simulink model "realtime"  (R2024b)
settings: Solver=VariableStepAuto  StartTime=0.0  StopTime=10.0  RelTol=1e-3
values from neighbouring files (symbols this model uses):
  C = Tc/(Tc+Ts)    [Observer_and_complementary_filter.m]    (also in init.m = @(q) [)
undefined symbols (not defined in the file or in its folder): denH, denHw, DiscIntNeverNeededParam, drv, dspblkCoreblockFVToolHelper, gbox, gcbh, integral, numH, numHw, sens, Ts, wheel
settings Model: Creator=lucag  LastModifiedBy=lucag

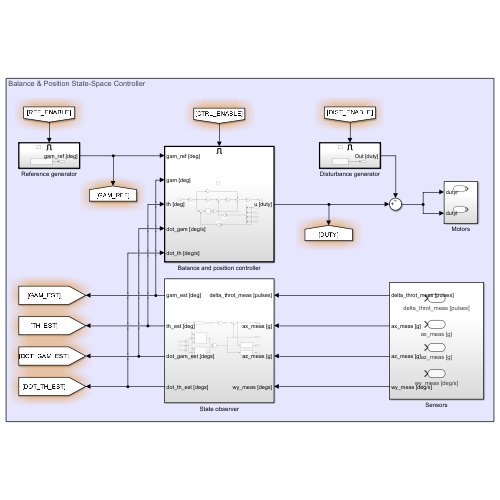
[thumbnail: Simulink's stored preview of the top-level diagram]
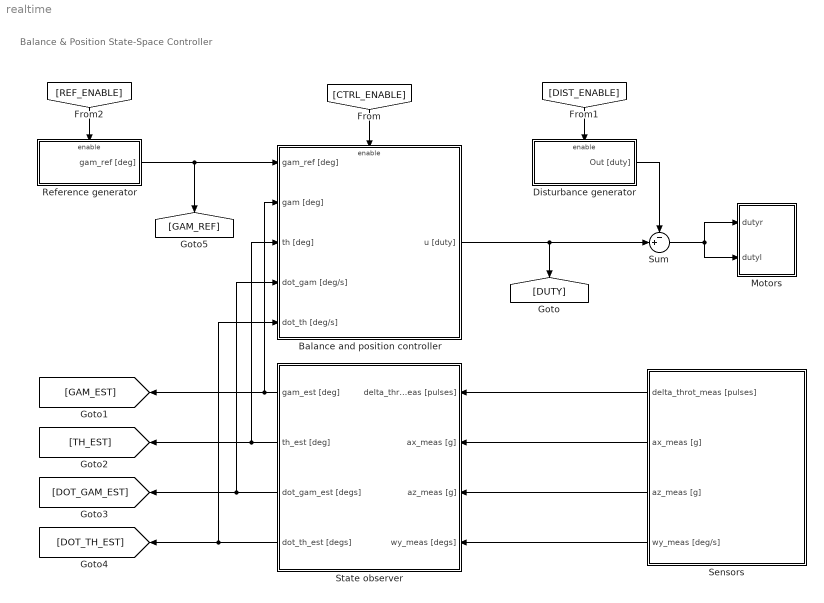
== system realtime ==
  note: Balance & Position State-Space Controller
  Balance and position controller : Subsystem  TreatAsAtomicUnit=on
  Disturbance generator : Subsystem  TreatAsAtomicUnit=on
  Motors : Subsystem
  Reference generator : Subsystem  TreatAsAtomicUnit=on
  Sensors : Subsystem
  State observer : Subsystem
  Sum : Sum  Inputs=-+|
  wires:
  [CTRL_ENABLE] -> Balance and position controller/Enable
  Balance and position controller/1(u [duty]) -> Sum/2, [DUTY]
  Disturbance generator/1(Out [duty]) -> Sum/1
  [DIST_ENABLE] -> Disturbance generator/Enable
  Sum/1 -> Motors/2(dutyl), Motors/1(dutyr)
  Sensors/1(delta_throt_meas [pulses]) -> State observer/1(delta_throt_meas [pulses])
  Sensors/2(ax_meas [g]) -> State observer/2(ax_meas [g])
  Sensors/3(az_meas [g]) -> State observer/3(az_meas [g])
  Sensors/4(wy_meas [deg/s]) -> State observer/4(wy_meas [degs])
  State observer/1(gam_est [deg]) -> [GAM_EST], Balance and position controller/2(gam [deg])
  State observer/2(th_est [deg]) -> [TH_EST], Balance and position controller/3(th [deg])
  State observer/3(dot_gam_est [degs]) -> Balance and position controller/4(dot_gam [deg/s]), [DOT_GAM_EST]
  State observer/4(dot_th_est [degs]) -> Balance and position controller/5(dot_th [deg/s]), [DOT_TH_EST]
  Reference generator/1(gam_ref [deg]) -> Balance and position controller/1(gam_ref [deg]), [GAM_REF]
  [REF_ENABLE] -> Reference generator/Enable

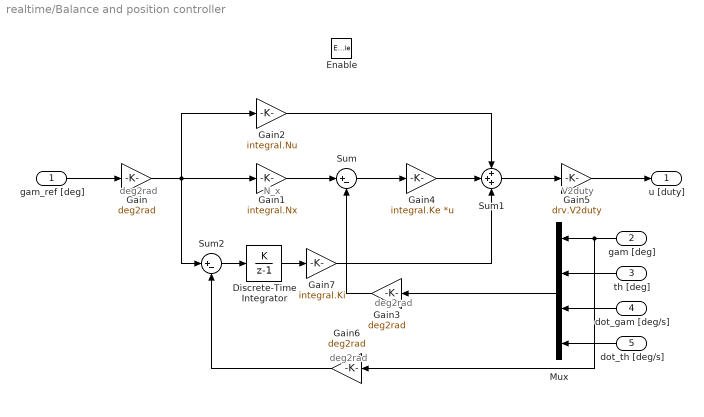
== system realtime/Balance and position controller ==
  note: deg2rad
  note: N_x
  note: V2duty
  note: deg2rad
  note: deg2rad
  gam_ref [deg] : Inport
  gam [deg] : Inport  Port=2
  th [deg] : Inport  Port=3
  dot_gam [deg/s] : Inport  Port=4
  dot_th [deg/s] : Inport  Port=5
  Enable : EnablePort
  Discrete-Time Integrator : DiscreteIntegrator  IntegratorMethod=Accumulation: Forward Euler  SampleTime=Ts  ICPrevOutput=DiscIntNeverNeededParam  ICPrevScaledInput=DiscIntNeverNeededParam
  Gain : Gain  Gain=deg2rad
  Gain1 : Gain  Gain=integral.Nx
  Gain2 : Gain  Gain=integral.Nu
  Gain3 : Gain  Gain=deg2rad
  Gain4 : Gain  Gain=integral.Ke  Multiplication=Matrix(K*u)
  Gain5 : Gain  Gain=drv.V2duty
  Gain6 : Gain  Gain=deg2rad
  Gain7 : Gain  Gain=integral.Ki
  Mux : Mux
  Sum : Sum  Inputs=|+-
  Sum1 : Sum  Inputs=+++
  Sum2 : Sum  Inputs=|+-
  u [duty] : Outport
  wires:
  dot_th [deg/s]/1 -> Mux/4
  Gain/1 -> Sum2/1, Gain2/1, Gain1/1
  Sum/1 -> Gain4/1
  Sum2/1 -> Discrete-Time Integrator/1
  gam_ref [deg]/1 -> Gain/1
  Gain7/1 -> Sum1/3
  Gain6/1 -> Sum2/2
  Discrete-Time Integrator/1 -> Gain7/1
  th [deg]/1 -> Mux/2
  Mux/1 -> Gain3/1
  Gain1/1 -> Sum/1
  Gain4/1 -> Sum1/2
  Sum1/1 -> Gain5/1
  gam [deg]/1 -> Gain6/1, Mux/1
  Gain5/1 -> u [duty]/1
  Gain2/1 -> Sum1/1
  Gain3/1 -> Sum/2
  dot_gam [deg/s]/1 -> Mux/3

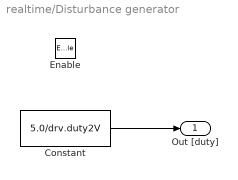
== system realtime/Disturbance generator ==
  Enable : EnablePort
  Constant : Constant  Value=5.0/drv.duty2V
  Out [duty] : Outport
  wires:
  Constant/1 -> Out [duty]/1

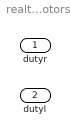
== system realtime/Motors ==
  dutyr : Inport
  dutyl : Inport  Port=2

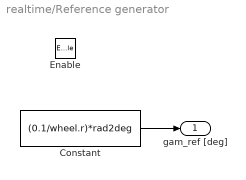
== system realtime/Reference generator ==
  Enable : EnablePort
  Constant : Constant  Value=(0.1/wheel.r)*rad2deg
  gam_ref [deg] : Outport
  wires:
  Constant/1 -> gam_ref [deg]/1

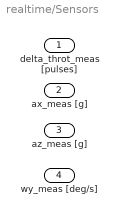
== system realtime/Sensors ==
  delta_throt_meas [pulses] : Outport
  ax_meas [g] : Outport  Port=2
  az_meas [g] : Outport  Port=3
  wy_meas [deg/s] : Outport  Port=4

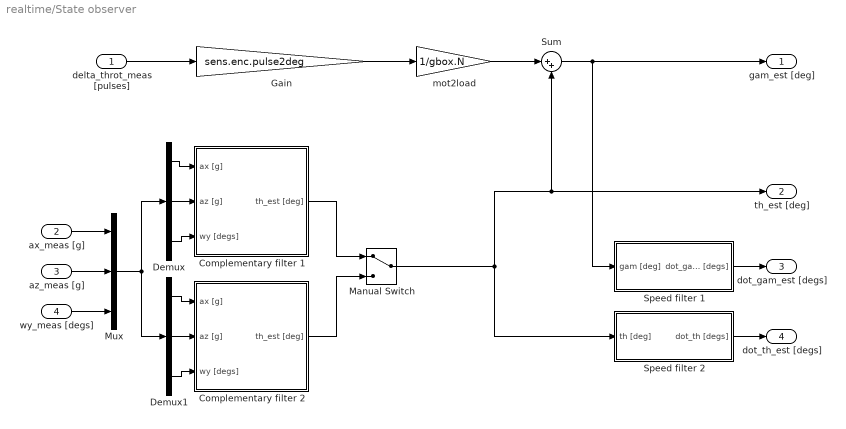
== system realtime/State observer ==
  delta_throt_meas [pulses] : Inport
  ax_meas [g] : Inport  Port=2
  az_meas [g] : Inport  Port=3
  wy_meas [degs] : Inport  Port=4
  Complementary filter 1 : Subsystem
  Complementary filter 2 : Subsystem
  Demux : Demux  Outputs=3
  Demux1 : Demux  Outputs=3
  Gain : Gain  Gain=sens.enc.pulse2deg
  Manual Switch : ManualSwitch
  Mux : Mux  Inputs=3
  Speed filter 1 : Subsystem
  Speed filter 2 : Subsystem
  Sum : Sum  Inputs=|++
  mot2load : Gain  Gain=1/gbox.N
  gam_est [deg] : Outport
  th_est [deg] : Outport  Port=2
  dot_gam_est [degs] : Outport  Port=3
  dot_th_est [degs] : Outport  Port=4
  wires:
  delta_throt_meas [pulses]/1 -> Gain/1
  Gain/1 -> mot2load/1
  mot2load/1 -> Sum/1
  Sum/1 -> Speed filter 1/1(gam [deg]), gam_est [deg]/1
  Speed filter 1/1(dot_gam [degs]) -> dot_gam_est [degs]/1
  Speed filter 2/1(dot_th [degs]) -> dot_th_est [degs]/1
  ax_meas [g]/1 -> Mux/1
  az_meas [g]/1 -> Mux/2
  wy_meas [degs]/1 -> Mux/3
  Demux/1 -> Complementary filter 1/1(ax [g])
  Demux/3 -> Complementary filter 1/3(wy [degs])
  Demux/2 -> Complementary filter 1/2(az [g])
  Demux1/2 -> Complementary filter 2/2(az [g])
  Demux1/1 -> Complementary filter 2/1(ax [g])
  Demux1/3 -> Complementary filter 2/3(wy [degs])
  Mux/1 -> Demux/1, Demux1/1
  Complementary filter 1/1(th_est [deg]) -> Manual Switch/1
  Complementary filter 2/1(th_est [deg]) -> Manual Switch/2
  Manual Switch/1 -> Sum/2, th_est [deg]/1, Speed filter 2/1(th [deg])

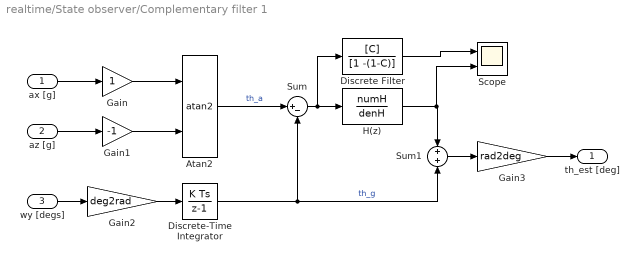
== system realtime/State observer/Complementary filter 1 ==
  ax [g] : Inport
  az [g] : Inport  Port=2
  wy [degs] : Inport  Port=3
  Atan2 : Trigonometry  Operator=atan2
  Discrete Filter : DiscreteFilter  LoadFcn=dspblkCoreblockFVToolHelper(gcbh,'load');  Numerator=[C]  Denominator=[1 -(1-C)]
      settings: CopyFcn=dspblkCoreblockFVToolHelper(gcbh,'copy');  DeleteFcn=dspblkCoreblockFVToolHelper(gcbh,'close');  ModelCloseFcn=dspblkCoreblockFVToolHelper(gcbh,'close');  PreSaveFcn=dspblkCoreblockFVToolHelper(gcbh,'presave');  PostSaveFcn=dspblkCoreblockFVToolHelper(gcbh,'postsave');  CloseFcn=dspblkCoreblockFVToolHelper(gcbh,'close');
  Discrete-Time Integrator : DiscreteIntegrator  SampleTime=Ts  ICPrevOutput=DiscIntNeverNeededParam  ICPrevScaledInput=DiscIntNeverNeededParam
  Gain : Gain
  Gain1 : Gain  Gain=-1
  Gain2 : Gain  Gain=deg2rad
  Gain3 : Gain  Gain=rad2deg
  H(z) : DiscreteTransferFcn  Numerator=numH  Denominator=denH
  Scope : Scope  NumInputPorts=2
  Sum : Sum  Inputs=|+-
  Sum1 : Sum  Inputs=+|+
  th_est [deg] : Outport
  wires:
  ax [g]/1 -> Gain/1
  az [g]/1 -> Gain1/1
  Gain/1 -> Atan2/1
  Gain1/1 -> Atan2/2
  Atan2/1 -> Sum/1  "th_a"
  wy [degs]/1 -> Gain2/1
  Gain2/1 -> Discrete-Time Integrator/1
  Discrete-Time Integrator/1 -> Sum1/2, Sum/2  "th_g"
  Sum/1 -> Discrete Filter/1, H(z)/1
  H(z)/1 -> Scope/2, Sum1/1
  Sum1/1 -> Gain3/1
  Gain3/1 -> th_est [deg]/1
  Discrete Filter/1 -> Scope/1

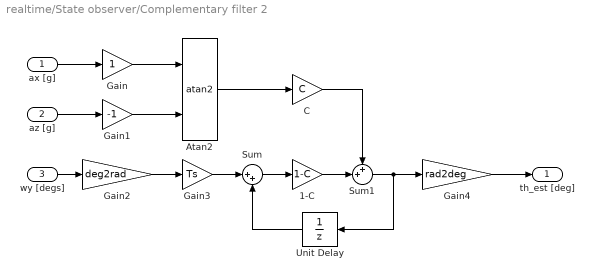
== system realtime/State observer/Complementary filter 2 ==
  ax [g] : Inport
  az [g] : Inport  Port=2
  wy [degs] : Inport  Port=3
  1-C : Gain  Gain=1-C
  Atan2 : Trigonometry  Operator=atan2
  C : Gain  Gain=C
  Gain : Gain
  Gain1 : Gain  Gain=-1
  Gain2 : Gain  Gain=deg2rad
  Gain3 : Gain  Gain=Ts
  Gain4 : Gain  Gain=rad2deg
  Sum : Sum  Inputs=|++
  Sum1 : Sum  Inputs=++|
  Unit Delay : UnitDelay  SampleTime=-1  HasFrameUpgradeWarning=on
  th_est [deg] : Outport
  wires:
  Gain/1 -> Atan2/1
  az [g]/1 -> Gain1/1
  Gain1/1 -> Atan2/2
  ax [g]/1 -> Gain/1
  Atan2/1 -> C/1
  wy [degs]/1 -> Gain2/1
  Gain2/1 -> Gain3/1
  Gain3/1 -> Sum/1
  Sum/1 -> 1-C/1
  C/1 -> Sum1/1
  1-C/1 -> Sum1/2
  Sum1/1 -> Unit Delay/1, Gain4/1
  Unit Delay/1 -> Sum/2
  Gain4/1 -> th_est [deg]/1

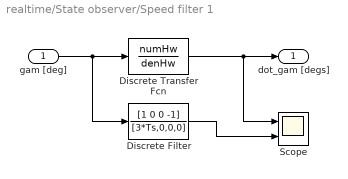
== system realtime/State observer/Speed filter 1 ==
  gam [deg] : Inport
  Discrete Transfer Fcn : DiscreteTransferFcn  Numerator=numHw  Denominator=denHw
  Discrete Filter : DiscreteFilter  LoadFcn=dspblkCoreblockFVToolHelper(gcbh,'load');  Numerator=[1 0 0 -1]  Denominator=[3*Ts,0,0,0]  SampleTime=Ts
      settings: CopyFcn=dspblkCoreblockFVToolHelper(gcbh,'copy');  DeleteFcn=dspblkCoreblockFVToolHelper(gcbh,'close');  ModelCloseFcn=dspblkCoreblockFVToolHelper(gcbh,'close');  PreSaveFcn=dspblkCoreblockFVToolHelper(gcbh,'presave');  PostSaveFcn=dspblkCoreblockFVToolHelper(gcbh,'postsave');  CloseFcn=dspblkCoreblockFVToolHelper(gcbh,'close');
  Scope : Scope  NumInputPorts=2
  dot_gam [degs] : Outport
  wires:
  gam [deg]/1 -> Discrete Filter/1, Discrete Transfer Fcn/1
  Discrete Transfer Fcn/1 -> Scope/1, dot_gam [degs]/1
  Discrete Filter/1 -> Scope/2

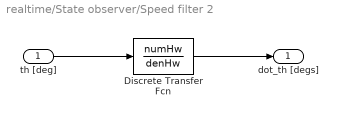
== system realtime/State observer/Speed filter 2 ==
  th [deg] : Inport
  Discrete Transfer Fcn : DiscreteTransferFcn  Numerator=numHw  Denominator=denHw
  dot_th [degs] : Outport
  wires:
  th [deg]/1 -> Discrete Transfer Fcn/1
  Discrete Transfer Fcn/1 -> dot_th [degs]/1
